simulink model "Pong3D"  (R2016b)
settings: Solver=ode45  StartTime=0.0  StopTime=10.0  FixedStep=0.001  MaxStep=updateFrequency  RelTol=1e-3  EnableMultiTasking=on
values from neighbouring files (symbols this model uses):
  Ball = struct(B_field1,B_value1,B_field2,B_value2,B_field3,B_value3,     B_field4,B_value4,B_field5,B_value5)    [PingPongStructs6DOF.m]
  Contact_Forces = struct(CF_field1,CF_value1,CF_field2,CF_value2,CF_field3,CF_value3)    [PingPongStructs6DOF.m]
  g = 9.81    [PingPongStructs6DOF.m]
  m = V(2)/V(1)    [AIPlayer.m]
  Net = struct(N_field1,N_value1)    [PingPongStructs6DOF.m]
  Robot1 = struct(R1_field1,R1_value1,R1_field2,R1_value2,R1_field3,R1_value3,     R1_field4,R1_value4, R1_field5,R1_value5,R1_field6,R1_value6,     R1_field7,R1_value7,R1_field8,R1_value8,R1_field9,R1_value9,R1_field10,R1_value10,     R1_field11,R1_value11,R1_field12,R1_value12)    [PingPongStructs6DOF.m]
  Robot2 = struct(R2_field1,R2_value1,R2_field2,R2_value2,R2_field3,R2_value3,     R2_field4, R2_value4, R2_field5,R2_value5,R2_field6,R2_value6,     R2_field7, R2_value7, R2_field8, R2_value8, R2_field9, R2_value9, R2_field10, R2_value10,     R2_field11, R2_value11, R2_field12, R2_value12)    [PingPongStructs6DOF.m]
  Table = struct(T_field1,T_value1,T_field2,T_value2)    [PingPongStructs6DOF.m]
undefined symbols (not defined in the file or in its folder): X, Y, Z
libraries: sm_lib x120, nesl_utility x55, fl_lib x48, Contact_Forces_Lib x4, Parts_Lib x3
(part 1 of 5)
settings Model: Creator=philipp  LastModifiedBy=philipp
settings DataIOCC: SaveFormat=Structure
settings OptimizationCC: LifeSpan=inf
settings DebuggingCC: SFUnexpectedBacktrackingDiag=warning  SFNoUnconditionalDefaultTransitionDiag=warning  SFExecutionAtInitializationDiag=none
settings HardwareCC: ProdBitPerSizeT=32  ProdBitPerPtrDiffT=32  ProdWordSize=32  ProdHWDeviceType=Specified
settings GRTTargetCC: TargetLangStandard=C89/C90 (ANSI)  GeneratePreprocessorConditionals=Disable all
settings ConfigComp: CovMetricSettings=dw  CovHtmlReporting=on  CovSaveCumulativeToWorkspaceVar=on  CovSaveSingleToWorkspaceVar=on  CovExternalEMLEnable=off
settings DiagnosticsConfigSet: SimMechanicsRigidlyBoundBlock=warning

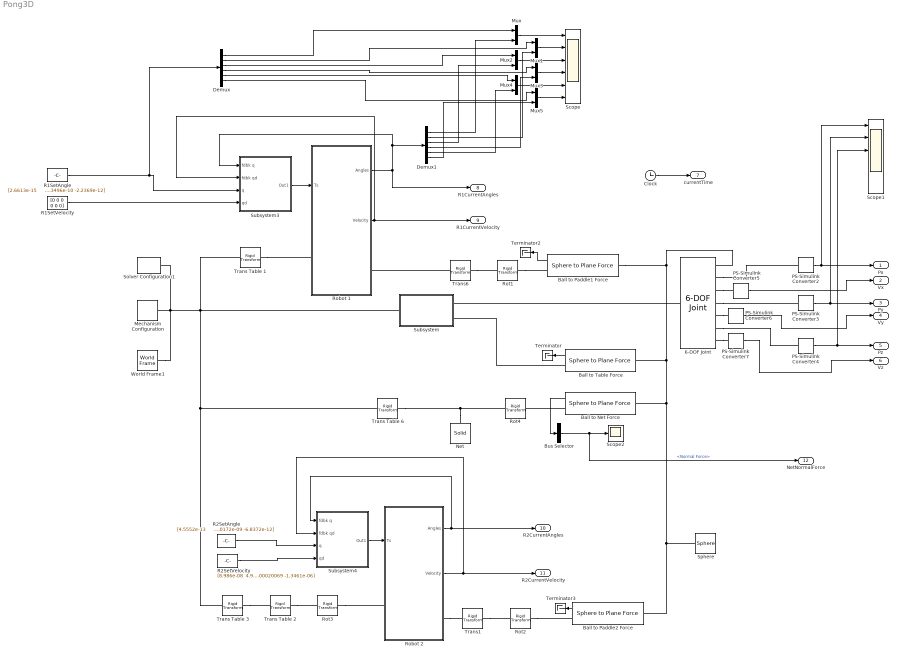
== system Pong3D ==
  6-DOF Joint : sm_lib/Joints/6-DOF Joint  SenseConstraintForce=off  SenseConstraintForceX=off  SenseConstraintForceY=off  SenseConstraintForceZ=off  SenseConstraintTorque=off  SenseConstraintTorqueX=off  SenseConstraintTorqueY=off  SenseConstraintTorqueZ=off  SenseTotalForce=off  SenseTotalForceX=off  SenseTotalForceY=off  SenseTotalForceZ=off  SenseTotalTorque=off  SenseTotalTorqueX=off  SenseTotalTorqueY=off  SenseTotalTorqueZ=off  CompositeWrenchDir=FollowerOnBase  CompositeWrenchFrame=BaseFrame  PxEquilibriumPosition=0  PxEquilibriumPositionUnits=m  PxSpringStiffness=0  PxSpringStiffnessUnits=N/m  PxDampingCoefficient=0  PxDampingCoefficientUnits=N/(m/s)  PxTorqueActuationMode=NoTorque  PxMotionActuationMode=ComputedMotion  PxSensePosition=on  PxSenseVelocity=on  PxSenseAcceleration=off  PxSenseTorqueForce=off  PxPositionTargetSpecify=on  PxPositionTargetPriority=High  PxPositionTargetValue=Ball.Initial_Position(1)  PxPositionTargetValueUnits=m  PxVelocityTargetSpecify=on  PxVelocityTargetPriority=High  PxVelocityTargetValue=Ball.Initial_Velocity(1)  PxVelocityTargetValueUnits=m/s  PyEquilibriumPosition=0  PyEquilibriumPositionUnits=m  PySpringStiffness=0  PySpringStiffnessUnits=N/m  PyDampingCoefficient=0  PyDampingCoefficientUnits=N/(m/s)  PyTorqueActuationMode=NoTorque  PyMotionActuationMode=ComputedMotion  PySensePosition=on  PySenseVelocity=on  PySenseAcceleration=off  PySenseTorqueForce=off  PyPositionTargetSpecify=on  PyPositionTargetPriority=High  PyPositionTargetValue=Ball.Initial_Position(2)  PyPositionTargetValueUnits=m  PyVelocityTargetSpecify=on  PyVelocityTargetPriority=High  PyVelocityTargetValue=Ball.Initial_Velocity(2)  PyVelocityTargetValueUnits=m/s  PzEquilibriumPosition=0  PzEquilibriumPositionUnits=m  PzSpringStiffness=0  PzSpringStiffnessUnits=N/m  PzDampingCoefficient=0  PzDampingCoefficientUnits=N/(m/s)  PzTorqueActuationMode=NoTorque  PzMotionActuationMode=ComputedMotion  PzSensePosition=on  PzSenseVelocity=on  PzSenseAcceleration=off  PzSenseTorqueForce=off  PzPositionTargetSpecify=on  PzPositionTargetPriority=High  PzPositionTargetValue=Ball.Initial_Position(3)  PzPositionTargetValueUnits=m  PzVelocityTargetSpecify=on  PzVelocityTargetPriority=High  PzVelocityTargetValue=Ball.Initial_Velocity(3)  PzVelocityTargetValueUnits=m/s  SphDefPosRotationMethod=None  SphDefPosRotationAngleUnits=deg  SphDefPosRotationStandardAxis=+Z  SphDefPosRotationAngle=0.0  SphDefPosRotationArbitraryAxis=[0 0 1]  SphDefPosFollAlignAxisA=+X  SphDefPosBaseAlignAxisA=+Y  SphDefPosFollAlignAxisB=+Y  SphDefPosBaseAlignAxisB=+Z  SphDefPosRotationSequenceAxes=FollowerAxes  SphDefPosRotationSequence=XYX  SphDefPosRotationSequenceAngles=[0 0 0]  SphDefPosRotationSequenceAnglesUnits=deg  SphDefPosRotationMatrix=[1 0 0; 0 1 0; 0 0 1]  SphEqPosRotationMethod=None  SphEqPosRotationAngleUnits=deg  SphEqPosRotationStandardAxis=+Z  SphEqPosRotationAngle=0.0  SphEqPosRotationArbitraryAxis=[0 0 1]  SphEqPosFollAlignAxisA=+X  SphEqPosBaseAlignAxisA=+Y  SphEqPosFollAlignAxisB=+Y  SphEqPosBaseAlignAxisB=+Z  SphEqPosRotationSequenceAxes=FollowerAxes  SphEqPosRotationSequence=XYX  SphEqPosRotationSequenceAngles=[0 0 0]  SphEqPosRotationSequenceAnglesUnits=deg  SphEqPosRotationMatrix=[1 0 0; 0 1 0; 0 0 1]  SphSpringStiffness=0  SphSpringStiffnessUnits=N*m/deg  SphDampingCoefficient=0  SphDampingCoefficientUnits=N*m/(deg/s)  SphActuateTorqueX=off  SphActuateTorqueY=off  SphActuateTorqueZ=off  SphActuateTorque=off  SphTorqueActuationMode=NoTorque  SphMotionActuationMode=ComputedMotion  SphActuationFrame=BaseFrame  SphSensePosition=off  SphSenseVelocityX=off  SphSenseVelocityY=off  SphSenseVelocityZ=off  SphSenseVelocity=off  SphSenseAccelerationX=off  SphSenseAccelerationY=off  SphSenseAccelerationZ=off  SphSenseAcceleration=off  SphSenseTorqueX=off  SphSenseTorqueY=off  SphSenseTorqueZ=off  SphSenseTorqueForce=off  SphSensingFrame=BaseFrame  SphPositionTargetRotationMethod=None  SphPositionTargetRotationAngleUnits=deg  SphPositionTargetRotationStandardAxis=+Z  SphPositionTargetRotationAngle=0.0  SphPositionTargetRotationArbitraryAxis=[0 0 1]  SphPositionTargetFollAlignAxisA=+X  SphPositionTargetBaseAlignAxisA=+Y  SphPositionTargetFollAlignAxisB=+Y  SphPositionTargetBaseAlignAxisB=+Z  SphPositionTargetRotationSequenceAxes=FollowerAxes  SphPositionTargetRotationSequence=XYX  SphPositionTargetRotationSequenceAngles=[0 0 0]  SphPositionTargetRotationSequenceAnglesUnits=deg  SphPositionTargetRotationMatrix=[1 0 0; 0 1 0; 0 0 1]  SphPositionTargetSpecify=off  SphPositionTargetPriority=High  SphVelocityTargetValue=[0 0 0]  SphVelocityTargetValueUnits=rad/s  SphVelocityTargetSpecify=off  SphVelocityTargetPriority=High  SphVelocityTargetInFollowerFrame=on
  Ball to Net Force : Contact_Forces_Lib/3D/Sphere to Plane Force  sphere_rad=Ball.Radius  plane_lenx=Net.Dimensions(3)  plane_leny=Net.Dimensions(1)  plane_depth=Net.Dimensions(2)/2  force_law=Linear  k_contact=Contact_Forces.Ball_Net(1)  b_contact=Contact_Forces.Ball_Net(2)  pen_full_damp_F=1e-4  pen_exponent=1  custom_param_1=1  custom_param_2=1  friction_law=None  mu_kinetic=0.5  mu_static=0.7  v_thr=0.001
  Ball to Paddle1 Force : Contact_Forces_Lib/3D/Sphere to Plane Force  sphere_rad=Ball.Radius  plane_lenx=2*Robot1.Paddle(1)  plane_leny=2*Robot1.Paddle(1)  plane_depth=Robot1.Paddle(2)/2  force_law=Linear  k_contact=Contact_Forces.Ball_Paddle(1)  b_contact=Contact_Forces.Ball_Paddle(2)  pen_full_damp_F=1e-4  pen_exponent=1  custom_param_1=1  custom_param_2=1  friction_law=None  mu_kinetic=0.5  mu_static=0.7  v_thr=0.001
  Ball to Paddle2 Force : Contact_Forces_Lib/3D/Sphere to Plane Force  sphere_rad=Ball.Radius  plane_lenx=2*Robot2.Paddle(1)  plane_leny=2*Robot2.Paddle(1)  plane_depth=Robot2.Paddle(2)/2  force_law=Linear  k_contact=Contact_Forces.Ball_Paddle(1)  b_contact=Contact_Forces.Ball_Paddle(2)  pen_full_damp_F=1e-4  pen_exponent=1  custom_param_1=1  custom_param_2=1  friction_law=None  mu_kinetic=0.5  mu_static=0.7  v_thr=0.001
  Ball to Table Force : Contact_Forces_Lib/3D/Sphere to Plane Force  sphere_rad=Ball.Radius  plane_lenx=Table.Dimensions(1)  plane_leny=Table.Dimensions(2)  plane_depth=Table.Dimensions(3)/2  force_law=Linear  k_contact=Contact_Forces.Ball_Table(1)  b_contact=Contact_Forces.Ball_Table(2)  pen_full_damp_F=1e-4  pen_exponent=1  custom_param_1=1  custom_param_2=1  friction_law=None  mu_kinetic=0.5  mu_static=0.7  v_thr=0.001
  Bus Selector : BusSelector  OutputSignals=Normal Force
  Clock : Clock
  Demux : Demux  Outputs=6
  Demux1 : Demux  Outputs=6
  Mechanism Configuration : sm_lib/Utilities/Mechanism Configuration  UniformGravity=Constant  GravityVector=[0 0 -g]  GravityUnits=m/s^2  LinearizationDelta=0.001
  Mux{,1..5} (6 alike) : Mux  Inputs=2
  Net : sm_lib/Body Elements/Solid  InertiaType=CalculateFromGeometry  Mass=1  MassUnits=kg  CenterOfMass=[0 0 0]  CenterOfMassUnits=m  MomentsOfInertia=[1 1 1]  MomentsOfInertiaUnits=kg*m^2  ProductsOfInertia=[0 0 0]  ProductsOfInertiaUnits=kg*m^2  DensityBased=on  Density=Net.Dimensions(4)  DensityUnits=kg/(m^3)  DoExposeReferenceFrame=on  SerializedFrames=<Frames/>  GraphicType=FromGeometry  MarkerShape=Sphere  MarkerSize=10  MarkerSizeUnits=m  GraphicVisPropType=SimpleVisualProperties  GraphicDiffuseColor=[1.0 1.0 1.0]  GraphicSpecularColor=[0.5 0.5 0.5 1.0]  GraphicAmbientColor=[0.15 0.15 0.15 1.0]  GraphicEmissiveColor=[0.0 0.0 0.0 1.0]  GraphicShininess=75  GraphicOpacity=1.0  GeometryShape=Brick  RectangleSize=[1 1]  RectangleSizeUnits=m  BrickDimensions=[Net.Dimensions(2) Net.Dimensions(1) Net.Dimensions(3)]  BrickDimensionUnits=m  CylinderRadius=1  CylinderRadiusUnits=m  CylinderLength=1  CylinderLengthUnits=m  SphereRadius=1  SphereRadiusUnits=m  EllipsoidRadii=[1 1 1]  EllipsoidRadiiUnits=m  ExtrusionCrossSection=[1 1; -1 1; -1 -1; 1 -1]  ExtrusionCrossSectionUnits=m  ExtrusionLength=1  ExtrusionLengthUnits=m  PolygonNumSides=3  PolygonOuterRadius=1  PolygonOuterRadiusUnits=m  ExtGeomFileType=STL  ExtGeomFileUnits=m  RevolutionCrossSection=[1 1; 1 -1; 2 -1; 2 1]  RevolutionCrossSectionUnits=m  RevolutionExtent=Full  RevolutionAngle=180  RevolutionAngleUnits=deg
  PS-Simulink Converter{2..7} (6 alike) : nesl_utility/PS-Simulink Converter  PhysicalDomain=network_engine_domain  SubClassName=ps_output  LeftPortType=input  RightPortType=output  PseudoPeriodic=off  Frequencies=[]  Unit=1  AffineConversion=off
  R1SetAngle : Constant  Value="[2.6613e-15      1.5708 -1.8519e-10  2.2643e-12  3.3496e-10 -2.2369e-12]"
  R1SetVelocity : Constant  Value="[0  0  0  0  0  0]"
  R2SetAngle : Constant  Value="[4.5552e-13      1.5708  -5.714e-10  6.9506e-12  1.0172e-09 -6.8372e-12]"
  R2SetVelocity : Constant  Value="[8.986e-08  4.9161e-06 -0.00011274  1.3713e-06  0.00020069 -1.3461e-06]"
  Robot 1 : Subsystem
  Robot 2 : Subsystem
  Rot1 : sm_lib/Frames and Transforms/Rigid Transform  TranslationMethod=None  TranslationStandardOffset=0  TranslationLengthUnit=m  TranslationStandardAxis=+Z  TranslationCartesianOffset=[0 0 0]  TranslationROffset=0  TranslationROffsetUnits=m  TranslationZOffset=0  TranslationZOffsetUnits=m  TranslationThetaOffset=0  TranslationThetaOffsetUnits=deg  RotationMethod=StandardAxis  RotationAngleUnits=deg  RotationStandardAxis=-Y  RotationAngle=90  RotationArbitraryAxis=[0 0 1]  FollAlignAxisA=+X  BaseAlignAxisA=+Y  FollAlignAxisB=+Y  BaseAlignAxisB=+Z  RotationSequenceAxes=FollowerAxes  RotationSequence=XYX  RotationSequenceAngles=[0 0 0]  RotationSequenceAnglesUnits=deg  RotationMatrix=[1 0 0; 0 1 0; 0 0 1]
      settings: AttributesFormatString=|
      | %<RotationAngle> %<RotationAngleUnits>
      | about %<RotationStandardAxis>
  Rot2 : sm_lib/Frames and Transforms/Rigid Transform  TranslationMethod=None  TranslationStandardOffset=0  TranslationLengthUnit=m  TranslationStandardAxis=+Z  TranslationCartesianOffset=[0 0 0]  TranslationROffset=0  TranslationROffsetUnits=m  TranslationZOffset=0  TranslationZOffsetUnits=m  TranslationThetaOffset=0  TranslationThetaOffsetUnits=deg  RotationMethod=StandardAxis  RotationAngleUnits=deg  RotationStandardAxis=-Y  RotationAngle=90  RotationArbitraryAxis=[0 0 1]  FollAlignAxisA=+X  BaseAlignAxisA=+Y  FollAlignAxisB=+Y  BaseAlignAxisB=+Z  RotationSequenceAxes=FollowerAxes  RotationSequence=XYX  RotationSequenceAngles=[0 0 0]  RotationSequenceAnglesUnits=deg  RotationMatrix=[1 0 0; 0 1 0; 0 0 1]
      settings: AttributesFormatString=|
      | %<RotationAngle> %<RotationAngleUnits>
      | about %<RotationStandardAxis>
  Rot3 : sm_lib/Frames and Transforms/Rigid Transform  TranslationMethod=None  TranslationStandardOffset=0  TranslationLengthUnit=m  TranslationStandardAxis=+Z  TranslationCartesianOffset=[0 0 0]  TranslationROffset=0  TranslationROffsetUnits=m  TranslationZOffset=0  TranslationZOffsetUnits=m  TranslationThetaOffset=0  TranslationThetaOffsetUnits=deg  RotationMethod=StandardAxis  RotationAngleUnits=deg  RotationStandardAxis=+Z  RotationAngle=180  RotationArbitraryAxis=[0 0 1]  FollAlignAxisA=+X  BaseAlignAxisA=+Y  FollAlignAxisB=+Y  BaseAlignAxisB=+Z  RotationSequenceAxes=FollowerAxes  RotationSequence=XYX  RotationSequenceAngles=[0 0 0]  RotationSequenceAnglesUnits=deg  RotationMatrix=[1 0 0; 0 1 0; 0 0 1]
      settings: AttributesFormatString=|
      | %<RotationAngle> %<RotationAngleUnits>
      | about %<RotationStandardAxis>
  Rot4 : sm_lib/Frames and Transforms/Rigid Transform  TranslationMethod=None  TranslationStandardOffset=0  TranslationLengthUnit=m  TranslationStandardAxis=+Z  TranslationCartesianOffset=[0 0 0]  TranslationROffset=0  TranslationROffsetUnits=m  TranslationZOffset=0  TranslationZOffsetUnits=m  TranslationThetaOffset=0  TranslationThetaOffsetUnits=deg  RotationMethod=StandardAxis  RotationAngleUnits=deg  RotationStandardAxis=-Y  RotationAngle=90  RotationArbitraryAxis=[0 0 1]  FollAlignAxisA=+X  BaseAlignAxisA=+Y  FollAlignAxisB=+Y  BaseAlignAxisB=+Z  RotationSequenceAxes=FollowerAxes  RotationSequence=XYX  RotationSequenceAngles=[0 0 0]  RotationSequenceAnglesUnits=deg  RotationMatrix=[1 0 0; 0 1 0; 0 0 1]
      settings: AttributesFormatString=|
      | %<RotationAngle> %<RotationAngleUnits>
      | about %<RotationStandardAxis>
  Scope : Scope  NumInputPorts=6
  Scope1 : Scope  NumInputPorts=6
  Scope2 : Scope
  Solver Configuration1 : nesl_utility/Solver Configuration  PhysicalDomain=network_engine_domain  SubClassName=solver  LeftPortType=input  RightPortType=generic  Accelerate=off  Tones=[]  Harmonics=[]  SimulateNoise=off  Profile=off  UseLocalSampling=off  EnableSwitchedLinearOptims=on  FrequencyDomain=off  UseCCode=off  RelTol=0.001  AbsTol=1e-06  MinStep=1e-09  ToWorkspace=off  RevertToSquareIcSolve=off  NumHomotopyIterations=100  PhasorMode=off  PhasorModeNumHarmonics=1  OverrideAbsTol=off  DoDC=off  ResidualTolerance=1e-09  UseLocalSolver=off  LocalSolverChoice=NE_BACKWARD_EULER_ADVANCER  LocalSolverSampleTime=0.001  DoFixedCost=off  MaxNonlinIter=3  MaxModeIter=2  LinearAlgebra=Sparse  DelaysMemoryBudget=1024  AutomaticFiltering=on  FilteringTimeConstant=0.001
  Sphere : Parts_Lib/Sphere  Tag=CustomStyle  sph_radius=Ball.Radius  sph_density=Ball.Density  sph_color=white  sph_opacity=1  mark_type=Rings on center planes  arc_width=[40 50]  arc_angle=60  ring_width=5  ring_irad=0.95  mark_color=axes  mark_opacity=1  ring_opacity=0  arc_opacity=0
  Subsystem : Subsystem
  Subsystem3 : Subsystem
  Subsystem4 : Subsystem
  Terminator : Terminator
  Terminator2 : Terminator
  Terminator3 : Terminator
  Trans Table 1 : sm_lib/Frames and Transforms/Rigid Transform  TranslationMethod=StandardAxis  TranslationStandardOffset=-Table.Dimensions(1)/2-Robot1.Distance_Table(1)  TranslationLengthUnit=m  TranslationStandardAxis=+X  TranslationCartesianOffset=[0 0 0]  TranslationROffset=0  TranslationROffsetUnits=m  TranslationZOffset=0  TranslationZOffsetUnits=m  TranslationThetaOffset=0  TranslationThetaOffsetUnits=deg  RotationMethod=None  RotationAngleUnits=deg  RotationStandardAxis=+Z  RotationAngle=0.0  RotationArbitraryAxis=[0 0 1]  FollAlignAxisA=+X  BaseAlignAxisA=+Y  FollAlignAxisB=+Y  BaseAlignAxisB=+Z  RotationSequenceAxes=FollowerAxes  RotationSequence=XYX  RotationSequenceAngles=[0 0 0]  RotationSequenceAnglesUnits=deg  RotationMatrix=[1 0 0; 0 1 0; 0 0 1]
      settings: AttributesFormatString=|
      | %<TranslationStandardOffset> %<TranslationLengthUnit>
      | in %<TranslationStandardAxis>
  Trans Table 2 : sm_lib/Frames and Transforms/Rigid Transform  TranslationMethod=StandardAxis  TranslationStandardOffset=-Table.Dimensions(1)/2-Robot1.Distance_Table(1)  TranslationLengthUnit=m  TranslationStandardAxis=+X  TranslationCartesianOffset=[0 0 0]  TranslationROffset=0  TranslationROffsetUnits=m  TranslationZOffset=0  TranslationZOffsetUnits=m  TranslationThetaOffset=0  TranslationThetaOffsetUnits=deg  RotationMethod=None  RotationAngleUnits=deg  RotationStandardAxis=+Z  RotationAngle=0.0  RotationArbitraryAxis=[0 0 1]  FollAlignAxisA=+X  BaseAlignAxisA=+Y  FollAlignAxisB=+Y  BaseAlignAxisB=+Z  RotationSequenceAxes=FollowerAxes  RotationSequence=XYX  RotationSequenceAngles=[0 0 0]  RotationSequenceAnglesUnits=deg  RotationMatrix=[1 0 0; 0 1 0; 0 0 1]
      settings: AttributesFormatString=|
      | %<TranslationStandardOffset> %<TranslationLengthUnit>
      | in %<TranslationStandardAxis>
  Trans Table 3 : sm_lib/Frames and Transforms/Rigid Transform  TranslationMethod=StandardAxis  TranslationStandardOffset=Table.Dimensions(1)+Robot1.Distance_Table(1)+Robot2.Distance_Table(1)  TranslationLengthUnit=m  TranslationStandardAxis=+X  TranslationCartesianOffset=[0 0 0]  TranslationROffset=0  TranslationROffsetUnits=m  TranslationZOffset=0  TranslationZOffsetUnits=m  TranslationThetaOffset=0  TranslationThetaOffsetUnits=deg  RotationMethod=None  RotationAngleUnits=deg  RotationStandardAxis=+Z  RotationAngle=0.0  RotationArbitraryAxis=[0 0 1]  FollAlignAxisA=+X  BaseAlignAxisA=+Y  FollAlignAxisB=+Y  BaseAlignAxisB=+Z  RotationSequenceAxes=FollowerAxes  RotationSequence=XYX  RotationSequenceAngles=[0 0 0]  RotationSequenceAnglesUnits=deg  RotationMatrix=[1 0 0; 0 1 0; 0 0 1]
      settings: AttributesFormatString=|
      | %<TranslationStandardOffset> %<TranslationLengthUnit>
      | in %<TranslationStandardAxis>
  Trans Table 6 : sm_lib/Frames and Transforms/Rigid Transform  TranslationMethod=StandardAxis  TranslationStandardOffset=Table.Height+Net.Dimensions(3)/2  TranslationLengthUnit=m  TranslationStandardAxis=+Z  TranslationCartesianOffset=[0 0 0]  TranslationROffset=0  TranslationROffsetUnits=m  TranslationZOffset=0  TranslationZOffsetUnits=m  TranslationThetaOffset=0  TranslationThetaOffsetUnits=deg  RotationMethod=None  RotationAngleUnits=deg  RotationStandardAxis=+Z  RotationAngle=0.0  RotationArbitraryAxis=[0 0 1]  FollAlignAxisA=+X  BaseAlignAxisA=+Y  FollAlignAxisB=+Y  BaseAlignAxisB=+Z  RotationSequenceAxes=FollowerAxes  RotationSequence=XYX  RotationSequenceAngles=[0 0 0]  RotationSequenceAnglesUnits=deg  RotationMatrix=[1 0 0; 0 1 0; 0 0 1]
      settings: AttributesFormatString=|
      | %<TranslationStandardOffset> %<TranslationLengthUnit>
      | in %<TranslationStandardAxis>
  Trans1 : sm_lib/Frames and Transforms/Rigid Transform  TranslationMethod=StandardAxis  TranslationStandardOffset=Robot2.Paddle(1)  TranslationLengthUnit=m  TranslationStandardAxis=-Z  TranslationCartesianOffset=[0 0 0]  TranslationROffset=0  TranslationROffsetUnits=m  TranslationZOffset=0  TranslationZOffsetUnits=m  TranslationThetaOffset=0  TranslationThetaOffsetUnits=deg  RotationMethod=None  RotationAngleUnits=deg  RotationStandardAxis=+Z  RotationAngle=0.0  RotationArbitraryAxis=[0 0 1]  FollAlignAxisA=+X  BaseAlignAxisA=+Y  FollAlignAxisB=+Y  BaseAlignAxisB=+Z  RotationSequenceAxes=FollowerAxes  RotationSequence=XYX  RotationSequenceAngles=[0 0 0]  RotationSequenceAnglesUnits=deg  RotationMatrix=[1 0 0; 0 1 0; 0 0 1]
      settings: AttributesFormatString=|
      | %<TranslationStandardOffset> %<TranslationLengthUnit>
      | in %<TranslationStandardAxis>
  Trans6 : sm_lib/Frames and Transforms/Rigid Transform  TranslationMethod=StandardAxis  TranslationStandardOffset=Robot1.Paddle(1)  TranslationLengthUnit=m  TranslationStandardAxis=-Z  TranslationCartesianOffset=[0 0 0]  TranslationROffset=0  TranslationROffsetUnits=m  TranslationZOffset=0  TranslationZOffsetUnits=m  TranslationThetaOffset=0  TranslationThetaOffsetUnits=deg  RotationMethod=None  RotationAngleUnits=deg  RotationStandardAxis=+Z  RotationAngle=0.0  RotationArbitraryAxis=[0 0 1]  FollAlignAxisA=+X  BaseAlignAxisA=+Y  FollAlignAxisB=+Y  BaseAlignAxisB=+Z  RotationSequenceAxes=FollowerAxes  RotationSequence=XYX  RotationSequenceAngles=[0 0 0]  RotationSequenceAnglesUnits=deg  RotationMatrix=[1 0 0; 0 1 0; 0 0 1]
      settings: AttributesFormatString=|
      | %<TranslationStandardOffset> %<TranslationLengthUnit>
      | in %<TranslationStandardAxis>
  World Frame1 : sm_lib/Frames and Transforms/World Frame
  Px : Outport
  Vx : Outport  Port=2
  Py : Outport  Port=3
  Vy : Outport  Port=4
  Pz : Outport  Port=5
  Vz : Outport  Port=6
  currentTime : Outport  Port=7
  R1CurrentAngles : Outport  Port=8  PortDimensions=[1,6]
  R1CurrentVelocity : Outport  Port=9  PortDimensions=[1,6]
  R2CurrentAngles : Outport  Port=10  PortDimensions=[1,6]
  R2CurrentVelocity : Outport  Port=11  PortDimensions=[1,6]
  NetNormalForce : Outport  Port=12
  wires:
  Subsystem3/1(Out1) -> Robot 1/1(Ts)
  Subsystem4/1(Out1) -> Robot 2/1(Ts)
  Ball to Table Force/1 -> Terminator/1
  Ball to Net Force/1 -> Bus Selector/1
  Ball to Paddle1 Force/1 -> Terminator2/1
  Ball to Paddle2 Force/1 -> Terminator3/1
  PS-Simulink Converter2/1 -> Px/1, Scope1/1
  PS-Simulink Converter4/1 -> Scope1/3, Pz/1
  PS-Simulink Converter3/1 -> Py/1, Scope1/2
  PS-Simulink Converter6/1 -> Vy/1
  PS-Simulink Converter5/1 -> Vx/1
  PS-Simulink Converter7/1 -> Vz/1
  R1SetAngle/1 -> Demux/1, Subsystem3/3(q)
  Mux/1 -> Scope/1
  Mux1/1 -> Scope/2
  Mux2/1 -> Scope/3
  Mux3/1 -> Scope/4
  Mux4/1 -> Scope/5
  Demux/5 -> Mux4/1
  Mux5/1 -> Scope/6
  Demux/1 -> Mux/1
  Demux/2 -> Mux1/1
  Demux/3 -> Mux2/1
  Demux/4 -> Mux3/1
  Demux/6 -> Mux5/1
  Demux1/1 -> Mux/2
  Demux1/2 -> Mux1/2
  Demux1/3 -> Mux2/2
  Demux1/4 -> Mux3/2
  Demux1/5 -> Mux4/2
  Demux1/6 -> Mux5/2
  R2SetAngle/1 -> Subsystem4/3(q)
  R1SetVelocity/1 -> Subsystem3/4(qd)
  R2SetVelocity/1 -> Subsystem4/4(qd)
  Robot 1/2(Velocity) -> Subsystem3/2(fdbk qd), R1CurrentVelocity/1
  Robot 1/1(Angles) -> R1CurrentAngles/1, Demux1/1, Subsystem3/1(fdbk q)
  Robot 2/1(Angles) -> Subsystem4/1(fdbk q), R2CurrentAngles/1
  Robot 2/2(Velocity) -> Subsystem4/2(fdbk qd), R2CurrentVelocity/1
  Bus Selector/1 -> NetNormalForce/1, Scope2/1  "<Normal Force>"
  Clock/1 -> currentTime/1
  connections:
  Net/RConn1 -- Rot4/LConn1 -- Trans Table 6/RConn1
  6-DOF Joint/LConn1 -- Subsystem/RConn1
  World Frame1/RConn1 -- Subsystem/LConn1 -- Trans Table 1/LConn1 -- Trans Table 6/LConn1 -- Trans Table 3/LConn1 -- Solver Configuration1/RConn1 -- Mechanism Configuration/RConn1
  Ball to Table Force/RConn1 -- Subsystem/RConn2
  Ball to Paddle2 Force/LConn1 -- Ball to Paddle1 Force/LConn1 -- 6-DOF Joint/RConn1 -- Ball to Table Force/LConn1 -- Ball to Net Force/LConn1 -- Sphere/LConn1
  Trans6/LConn1 -- Robot 1/RConn1
  Robot 2/RConn1 -- Trans1/LConn1
  Rot3/RConn1 -- Robot 2/LConn1
  Trans Table 3/RConn1 -- Trans Table 2/LConn1
  6-DOF Joint/RConn2 -- PS-Simulink Converter2/LConn1
  6-DOF Joint/RConn3 -- PS-Simulink Converter5/LConn1
  6-DOF Joint/RConn4 -- PS-Simulink Converter3/LConn1
  6-DOF Joint/RConn6 -- PS-Simulink Converter4/LConn1
  6-DOF Joint/RConn5 -- PS-Simulink Converter6/LConn1
  6-DOF Joint/RConn7 -- PS-Simulink Converter7/LConn1
  Rot1/RConn1 -- Ball to Paddle1 Force/RConn1
  Trans6/RConn1 -- Rot1/LConn1
  Rot2/RConn1 -- Ball to Paddle2 Force/RConn1
  Trans1/RConn1 -- Rot2/LConn1
  Trans Table 1/RConn1 -- Robot 1/LConn1
  Trans Table 2/RConn1 -- Rot3/LConn1
  Ball to Net Force/RConn1 -- Rot4/RConn1

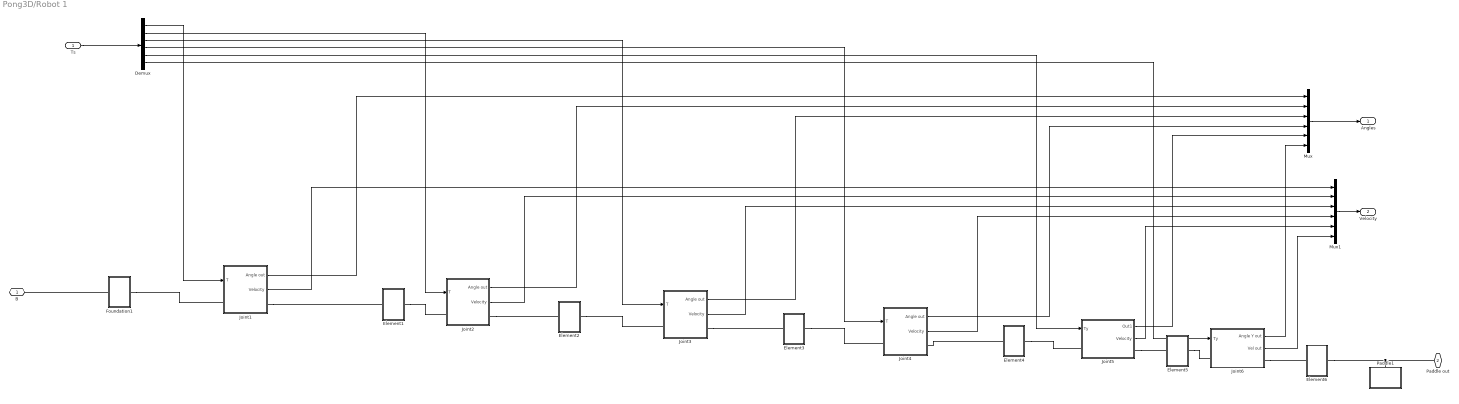
== system Pong3D/Robot 1 ==
  Ts : Inport
  Demux : Demux  Outputs=6
  Element1 : Subsystem
  Element2 : Subsystem
  Element3 : Subsystem
  Element4 : Subsystem
  Element5 : Subsystem
  Element6 : Subsystem
  Foundation1 : Subsystem
  Joint1 : Subsystem
  Joint2 : Subsystem
  Joint3 : Subsystem
  Joint4 : Subsystem
  Joint5 : Subsystem
  Joint6 : Subsystem
  Mux : Mux  Inputs=6
  Mux1 : Mux  Inputs=6
  Paddle1 : Subsystem
  B : PMIOPort  Port=1  Side=Left
  Paddle out : PMIOPort  Port=2  Side=Right
  Angles : Outport
  Velocity : Outport  Port=2
  wires:
  Joint6/1(Angle Y out) -> Mux/6
  Joint5/1(Out1) -> Mux/5
  Joint4/1(Angle out) -> Mux/4
  Joint3/1(Angle out) -> Mux/3
  Joint2/1(Angle out) -> Mux/2
  Joint1/1(Angle out) -> Mux/1
  Ts/1 -> Demux/1
  Demux/1 -> Joint1/1(T)
  Demux/2 -> Joint2/1(T)
  Demux/3 -> Joint3/1(T)
  Demux/4 -> Joint4/1(T)
  Demux/5 -> Joint5/1(Ty)
  Demux/6 -> Joint6/1(Ty)
  Joint6/2(Vel out) -> Mux1/6
  Mux/1 -> Angles/1
  Mux1/1 -> Velocity/1
  Joint5/2(Velocity) -> Mux1/5
  Joint4/2(Velocity) -> Mux1/4
  Joint3/2(Velocity) -> Mux1/3
  Joint2/2(Velocity) -> Mux1/2
  Joint1/2(Velocity) -> Mux1/1
  connections:
  Joint4/RConn1 -- Element4/LConn1
  Element3/RConn1 -- Joint4/LConn1
  Joint2/RConn1 -- Element2/LConn1
  Element1/RConn1 -- Joint2/LConn1
  Foundation1/RConn1 -- Joint1/LConn1
  Joint3/RConn1 -- Element3/LConn1
  Element4/RConn1 -- Joint5/LConn1
  Element5/RConn1 -- Joint6/LConn1
  Joint6/RConn1 -- Element6/LConn1
  Foundation1/LConn1 -- B/RConn1
  Joint1/RConn1 -- Element1/LConn1
  Element2/RConn1 -- Joint3/LConn1
  Joint5/RConn1 -- Element5/LConn1
  Element6/RConn1 -- Paddle out/RConn1 -- Paddle1/LConn1

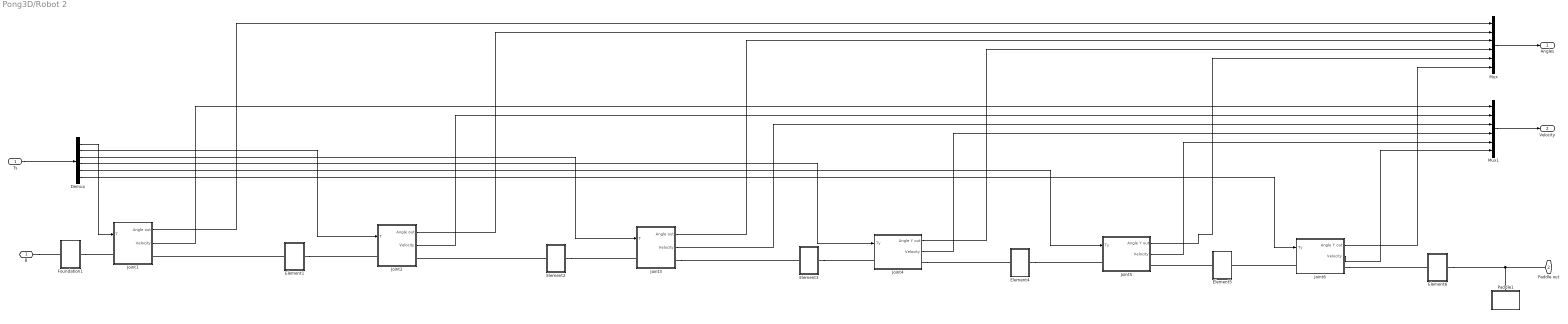
== system Pong3D/Robot 2 ==
  Ts : Inport
  Demux : Demux  Outputs=6
  Element1 : Subsystem
  Element2 : Subsystem
  Element3 : Subsystem
  Element4 : Subsystem
  Element5 : Subsystem
  Element6 : Subsystem
  Foundation1 : Subsystem
  Joint1 : Subsystem
  Joint2 : Subsystem
  Joint3 : Subsystem
  Joint4 : Subsystem
  Joint5 : Subsystem
  Joint6 : Subsystem
  Mux : Mux  Inputs=6
  Mux1 : Mux  Inputs=6
  Paddle1 : Subsystem
  B : PMIOPort  Port=1  Side=Left
  Paddle out : PMIOPort  Port=2  Side=Right
  Angles : Outport
  Velocity : Outport  Port=2
  wires:
  Ts/1 -> Demux/1
  Demux/1 -> Joint1/1(T)
  Demux/2 -> Joint2/1(T)
  Demux/3 -> Joint3/1(T)
  Demux/4 -> Joint4/1(Ty)
  Demux/5 -> Joint5/1(Ty)
  Demux/6 -> Joint6/1(Ty)
  Mux/1 -> Angles/1
  Joint6/1(Angle Y out) -> Mux/6
  Joint5/1(Angle Y out) -> Mux/5
  Joint4/1(Angle Y out) -> Mux/4
  Joint3/1(Angle out) -> Mux/3
  Joint2/1(Angle out) -> Mux/2
  Joint1/1(Angle out) -> Mux/1
  Mux1/1 -> Velocity/1
  Joint6/2(Velocity) -> Mux1/6
  Joint5/2(Velocity) -> Mux1/5
  Joint4/2(Velocity) -> Mux1/4
  Joint3/2(Velocity) -> Mux1/3
  Joint2/2(Velocity) -> Mux1/2
  Joint1/2(Velocity) -> Mux1/1
  connections:
  Element2/LConn1 -- Joint2/RConn1
  Element4/RConn1 -- Joint5/LConn1
  Element1/RConn1 -- Joint2/LConn1
  Element2/RConn1 -- Joint3/LConn1
  Element3/RConn1 -- Joint4/LConn1
  Element5/LConn1 -- Joint5/RConn1
  Element1/LConn1 -- Joint1/RConn1
  B/RConn1 -- Foundation1/LConn1
  Foundation1/RConn1 -- Joint1/LConn1
  Joint3/RConn1 -- Element3/LConn1
  Joint4/RConn1 -- Element4/LConn1
  Paddle out/RConn1 -- Element6/RConn1 -- Paddle1/LConn1
  Joint6/LConn1 -- Element5/RConn1
  Joint6/RConn1 -- Element6/LConn1

== system Pong3D/Subsystem ==
  Table : sm_lib/Body Elements/Solid  InertiaType=CalculateFromGeometry  Mass=1  MassUnits=kg  CenterOfMass=[0 0 0]  CenterOfMassUnits=m  MomentsOfInertia=[1 1 1]  MomentsOfInertiaUnits=kg*m^2  ProductsOfInertia=[0 0 0]  ProductsOfInertiaUnits=kg*m^2  DensityBased=on  Density=Table.Dimensions(4)  DensityUnits=kg/(m^3)  DoExposeReferenceFrame=on  SerializedFrames=<Frames/>  GraphicType=FromGeometry  MarkerShape=Sphere  MarkerSize=10  MarkerSizeUnits=m  GraphicVisPropType=SimpleVisualProperties  GraphicDiffuseColor=[0.0 0.4 0.4]  GraphicSpecularColor=[0.5 0.5 0.5 1.0]  GraphicAmbientColor=[0.15 0.15 0.15 1.0]  GraphicEmissiveColor=[0.0 0.0 0.0 1.0]  GraphicShininess=75  GraphicOpacity=1.0  GeometryShape=Brick  RectangleSize=[1 1]  RectangleSizeUnits=m  BrickDimensions=[Table.Dimensions(1) Table.Dimensions(2) Table.Dimensions(3)]  BrickDimensionUnits=m  CylinderRadius=0.05  CylinderRadiusUnits=m  CylinderLength=0.5  CylinderLengthUnits=m  SphereRadius=1  SphereRadiusUnits=m  EllipsoidRadii=[1 1 1]  EllipsoidRadiiUnits=m  ExtrusionCrossSection=[1 1; -1 1; -1 -1; 1 -1]  ExtrusionCrossSectionUnits=m  ExtrusionLength=1  ExtrusionLengthUnits=m  PolygonNumSides=3  PolygonOuterRadius=1  PolygonOuterRadiusUnits=m  ExtGeomFileType=STL  ExtGeomFileUnits=m  RevolutionCrossSection=[1 1; 1 -1; 2 -1; 2 1]  RevolutionCrossSectionUnits=m  RevolutionExtent=Full  RevolutionAngle=180  RevolutionAngleUnits=deg
  Trans Table 3 : sm_lib/Frames and Transforms/Rigid Transform  TranslationMethod=StandardAxis  TranslationStandardOffset=Table.Height-Table.Dimensions(3)/2  TranslationLengthUnit=m  TranslationStandardAxis=+Z  TranslationCartesianOffset=[0 0 0]  TranslationROffset=0  TranslationROffsetUnits=m  TranslationZOffset=0  TranslationZOffsetUnits=m  TranslationThetaOffset=0  TranslationThetaOffsetUnits=deg  RotationMethod=None  RotationAngleUnits=deg  RotationStandardAxis=+Z  RotationAngle=0.0  RotationArbitraryAxis=[0 0 1]  FollAlignAxisA=+X  BaseAlignAxisA=+Y  FollAlignAxisB=+Y  BaseAlignAxisB=+Z  RotationSequenceAxes=FollowerAxes  RotationSequence=XYX  RotationSequenceAngles=[0 0 0]  RotationSequenceAnglesUnits=deg  RotationMatrix=[1 0 0; 0 1 0; 0 0 1]
      settings: AttributesFormatString=|
      | %<TranslationStandardOffset> %<TranslationLengthUnit>
      | in %<TranslationStandardAxis>
  In : PMIOPort  Port=1  Side=Left
  Bottom : PMIOPort  Port=2  Side=Right
  Center_Table : PMIOPort  Port=3  Side=Right
  connections:
  Center_Table/RConn1 -- Trans Table 3/RConn1 -- Table/RConn1
  Bottom/RConn1 -- In/RConn1 -- Trans Table 3/LConn1

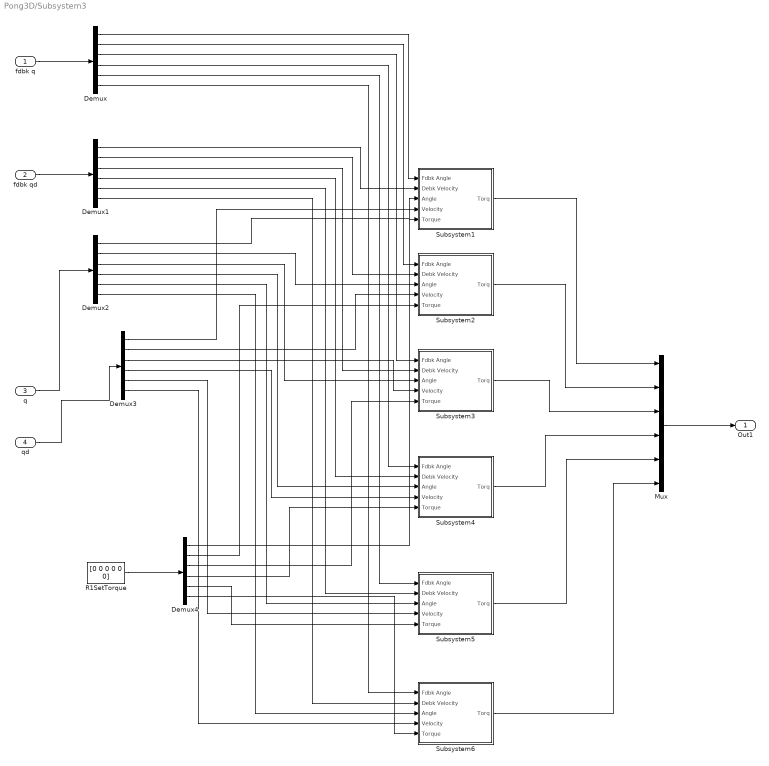
== system Pong3D/Subsystem3 ==
  fdbk q : Inport
  fdbk qd : Inport  Port=2
  q : Inport  Port=3
  qd : Inport  Port=4
  Demux{,1..4} (5 alike) : Demux  Outputs=6
  Mux : Mux  Inputs=6
  R1SetTorque : Constant  Value=[0 0 0 0 0 0]
  Subsystem1 : Subsystem
  Subsystem2 : Subsystem
  Subsystem3 : Subsystem
  Subsystem4 : Subsystem
  Subsystem5 : Subsystem
  Subsystem6 : Subsystem
  Out1 : Outport
  wires:
  q/1 -> Demux2/1
  qd/1 -> Demux3/1
  fdbk q/1 -> Demux/1
  Demux/1 -> Subsystem1/1(Fdbk Angle)
  Demux/2 -> Subsystem2/1(Fdbk Angle)
  Demux/3 -> Subsystem3/1(Fdbk Angle)
  Demux/4 -> Subsystem4/1(Fdbk Angle)
  Demux/5 -> Subsystem5/1(Fdbk Angle)
  Demux/6 -> Subsystem6/1(Fdbk Angle)
  fdbk qd/1 -> Demux1/1
  Demux1/1 -> Subsystem1/2(Debk Velocity)
  Demux1/2 -> Subsystem2/2(Debk Velocity)
  Demux1/3 -> Subsystem3/2(Debk Velocity)
  Demux1/4 -> Subsystem4/2(Debk Velocity)
  Demux1/5 -> Subsystem5/2(Debk Velocity)
  Demux1/6 -> Subsystem6/2(Debk Velocity)
  Demux2/1 -> Subsystem1/3(Angle)
  Demux2/2 -> Subsystem2/3(Angle)
  Demux2/3 -> Subsystem3/3(Angle)
  Demux2/4 -> Subsystem4/3(Angle)
  Demux2/5 -> Subsystem5/3(Angle)
  Demux2/6 -> Subsystem6/3(Angle)
  Demux3/1 -> Subsystem1/4(Velocity)
  Demux3/2 -> Subsystem2/4(Velocity)
  Demux3/3 -> Subsystem3/4(Velocity)
  Demux3/4 -> Subsystem4/4(Velocity)
  Demux3/5 -> Subsystem5/4(Velocity)
  Demux3/6 -> Subsystem6/4(Velocity)
  Demux4/1 -> Subsystem1/5(Torque)
  Demux4/2 -> Subsystem2/5(Torque)
  Demux4/3 -> Subsystem3/5(Torque)
  Demux4/4 -> Subsystem4/5(Torque)
  Demux4/5 -> Subsystem5/5(Torque)
  Demux4/6 -> Subsystem6/5(Torque)
  Subsystem1/1(Torq) -> Mux/1
  Subsystem2/1(Torq) -> Mux/2
  Subsystem3/1(Torq) -> Mux/3
  Subsystem4/1(Torq) -> Mux/4
  Subsystem5/1(Torq) -> Mux/5
  Subsystem6/1(Torq) -> Mux/6
  Mux/1 -> Out1/1
  R1SetTorque/1 -> Demux4/1

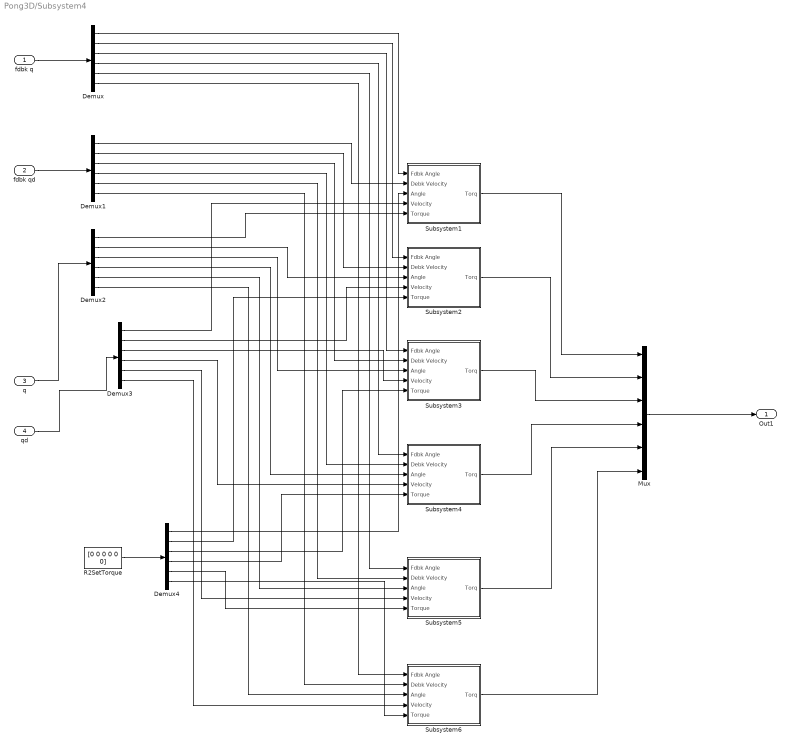
== system Pong3D/Subsystem4 ==
  fdbk q : Inport
  fdbk qd : Inport  Port=2
  q : Inport  Port=3
  qd : Inport  Port=4
  Demux{,1..4} (5 alike) : Demux  Outputs=6
  Mux : Mux  Inputs=6
  R2SetTorque : Constant  Value=[0 0 0 0 0 0]
  Subsystem1 : Subsystem
  Subsystem2 : Subsystem
  Subsystem3 : Subsystem
  Subsystem4 : Subsystem
  Subsystem5 : Subsystem
  Subsystem6 : Subsystem
  Out1 : Outport
  wires:
  Mux/1 -> Out1/1
  Subsystem6/1(Torq) -> Mux/6
  Subsystem5/1(Torq) -> Mux/5
  Subsystem4/1(Torq) -> Mux/4
  Subsystem3/1(Torq) -> Mux/3
  Subsystem2/1(Torq) -> Mux/2
  Subsystem1/1(Torq) -> Mux/1
  Demux4/6 -> Subsystem6/5(Torque)
  Demux4/5 -> Subsystem5/5(Torque)
  Demux4/4 -> Subsystem4/5(Torque)
  Demux4/3 -> Subsystem3/5(Torque)
  Demux4/2 -> Subsystem2/5(Torque)
  Demux4/1 -> Subsystem1/5(Torque)
  Demux3/6 -> Subsystem6/4(Velocity)
  Demux3/5 -> Subsystem5/4(Velocity)
  Demux3/4 -> Subsystem4/4(Velocity)
  Demux3/3 -> Subsystem3/4(Velocity)
  Demux3/2 -> Subsystem2/4(Velocity)
  Demux3/1 -> Subsystem1/4(Velocity)
  Demux2/6 -> Subsystem6/3(Angle)
  Demux2/5 -> Subsystem5/3(Angle)
  Demux2/4 -> Subsystem4/3(Angle)
  Demux2/3 -> Subsystem3/3(Angle)
  Demux2/2 -> Subsystem2/3(Angle)
  Demux2/1 -> Subsystem1/3(Angle)
  Demux1/6 -> Subsystem6/2(Debk Velocity)
  Demux1/5 -> Subsystem5/2(Debk Velocity)
  Demux1/4 -> Subsystem4/2(Debk Velocity)
  Demux1/3 -> Subsystem3/2(Debk Velocity)
  Demux1/2 -> Subsystem2/2(Debk Velocity)
  Demux1/1 -> Subsystem1/2(Debk Velocity)
  fdbk qd/1 -> Demux1/1
  Demux/6 -> Subsystem6/1(Fdbk Angle)
  Demux/5 -> Subsystem5/1(Fdbk Angle)
  Demux/4 -> Subsystem4/1(Fdbk Angle)
  Demux/3 -> Subsystem3/1(Fdbk Angle)
  Demux/2 -> Subsystem2/1(Fdbk Angle)
  Demux/1 -> Subsystem1/1(Fdbk Angle)
  fdbk q/1 -> Demux/1
  qd/1 -> Demux3/1
  q/1 -> Demux2/1
  R2SetTorque/1 -> Demux4/1

== system Pong3D/Robot 1/Element1 ==
  Rot1 : sm_lib/Frames and Transforms/Rigid Transform  TranslationMethod=None  TranslationStandardOffset=0  TranslationLengthUnit=m  TranslationStandardAxis=+Z  TranslationCartesianOffset=[0 0 0]  TranslationROffset=0  TranslationROffsetUnits=m  TranslationZOffset=0  TranslationZOffsetUnits=m  TranslationThetaOffset=0  TranslationThetaOffsetUnits=deg  RotationMethod=StandardAxis  RotationAngleUnits=deg  RotationStandardAxis=-Y  RotationAngle=90  RotationArbitraryAxis=[0 0 1]  FollAlignAxisA=+X  BaseAlignAxisA=+Y  FollAlignAxisB=+Y  BaseAlignAxisB=+Z  RotationSequenceAxes=FollowerAxes  RotationSequence=XYX  RotationSequenceAngles=[0 0 0]  RotationSequenceAnglesUnits=deg  RotationMatrix=[1 0 0; 0 1 0; 0 0 1]
      settings: AttributesFormatString=|
      | %<RotationAngle> %<RotationAngleUnits>
      | about %<RotationStandardAxis>
  Rot2 : sm_lib/Frames and Transforms/Rigid Transform  TranslationMethod=None  TranslationStandardOffset=0  TranslationLengthUnit=m  TranslationStandardAxis=+Z  TranslationCartesianOffset=[0 0 0]  TranslationROffset=0  TranslationROffsetUnits=m  TranslationZOffset=0  TranslationZOffsetUnits=m  TranslationThetaOffset=0  TranslationThetaOffsetUnits=deg  RotationMethod=StandardAxis  RotationAngleUnits=deg  RotationStandardAxis=+Y  RotationAngle=90  RotationArbitraryAxis=[0 0 1]  FollAlignAxisA=+X  BaseAlignAxisA=+Y  FollAlignAxisB=+Y  BaseAlignAxisB=+Z  RotationSequenceAxes=FollowerAxes  RotationSequence=XYX  RotationSequenceAngles=[0 0 0]  RotationSequenceAnglesUnits=deg  RotationMatrix=[1 0 0; 0 1 0; 0 0 1]
      settings: AttributesFormatString=|
      | %<RotationAngle> %<RotationAngleUnits>
      | about %<RotationStandardAxis>
  Rot4 : sm_lib/Frames and Transforms/Rigid Transform  TranslationMethod=None  TranslationStandardOffset=0  TranslationLengthUnit=m  TranslationStandardAxis=+Z  TranslationCartesianOffset=[0 0 0]  TranslationROffset=0  TranslationROffsetUnits=m  TranslationZOffset=0  TranslationZOffsetUnits=m  TranslationThetaOffset=0  TranslationThetaOffsetUnits=deg  RotationMethod=StandardAxis  RotationAngleUnits=deg  RotationStandardAxis=+X  RotationAngle=90  RotationArbitraryAxis=[0 0 1]  FollAlignAxisA=+X  BaseAlignAxisA=+Y  FollAlignAxisB=+Y  BaseAlignAxisB=+Z  RotationSequenceAxes=FollowerAxes  RotationSequence=XYX  RotationSequenceAngles=[0 0 0]  RotationSequenceAnglesUnits=deg  RotationMatrix=[1 0 0; 0 1 0; 0 0 1]
      settings: AttributesFormatString=|
      | %<RotationAngle> %<RotationAngleUnits>
      | about %<RotationStandardAxis>
  Solid2 : sm_lib/Body Elements/Solid  InertiaType=CalculateFromGeometry  Mass=Robot1.Element1(1)  MassUnits=kg  CenterOfMass=[0 0 0]  CenterOfMassUnits=m  MomentsOfInertia=[1 1 1]  MomentsOfInertiaUnits=kg*m^2  ProductsOfInertia=[0 0 0]  ProductsOfInertiaUnits=kg*m^2  DensityBased=off  Density=1000  DensityUnits=kg/(m^3)  DoExposeReferenceFrame=on  SerializedFrames=<Frames/>  GraphicType=FromGeometry  MarkerShape=Sphere  MarkerSize=10  MarkerSizeUnits=m  GraphicVisPropType=SimpleVisualProperties  GraphicDiffuseColor=[0.6 0.0 0.0]  GraphicSpecularColor=[0.5 0.5 0.5 1.0]  GraphicAmbientColor=[0.15 0.15 0.15 1.0]  GraphicEmissiveColor=[0.0 0.0 0.0 1.0]  GraphicShininess=75  GraphicOpacity=1.0  GeometryShape=FromFile  RectangleSize=[1 1]  RectangleSizeUnits=m  BrickDimensions=[1 1 1]  BrickDimensionUnits=m  CylinderRadius=1  CylinderRadiusUnits=m  CylinderLength=1  CylinderLengthUnits=m  SphereRadius=1  SphereRadiusUnits=m  EllipsoidRadii=[1 1 1]  EllipsoidRadiiUnits=m  ExtrusionCrossSection=[1 1; -1 1; -1 -1; 1 -1]  ExtrusionCrossSectionUnits=m  ExtrusionLength=1  ExtrusionLengthUnits=m  PolygonNumSides=3  PolygonOuterRadius=1  PolygonOuterRadiusUnits=m  ExtGeomFileType=STEP  ExtGeomFileName=./StepData_DHPara/Element1.stp  ExtGeomFileUnits=m  RevolutionCrossSection=[1 1; 1 -1; 2 -1; 2 1]  RevolutionCrossSectionUnits=m  RevolutionExtent=Full  RevolutionAngle=180  RevolutionAngleUnits=deg
  Trans2 : sm_lib/Frames and Transforms/Rigid Transform  TranslationMethod=StandardAxis  TranslationStandardOffset=Robot1.Element1(2)  TranslationLengthUnit=m  TranslationStandardAxis=+Z  TranslationCartesianOffset=[0 0 0]  TranslationROffset=0  TranslationROffsetUnits=m  TranslationZOffset=0  TranslationZOffsetUnits=m  TranslationThetaOffset=0  TranslationThetaOffsetUnits=deg  RotationMethod=None  RotationAngleUnits=deg  RotationStandardAxis=+Z  RotationAngle=0.0  RotationArbitraryAxis=[0 0 1]  FollAlignAxisA=+X  BaseAlignAxisA=+Y  FollAlignAxisB=+Y  BaseAlignAxisB=+Z  RotationSequenceAxes=FollowerAxes  RotationSequence=XYX  RotationSequenceAngles=[0 0 0]  RotationSequenceAnglesUnits=deg  RotationMatrix=[1 0 0; 0 1 0; 0 0 1]
      settings: AttributesFormatString=|
      | %<TranslationStandardOffset> %<TranslationLengthUnit>
      | in %<TranslationStandardAxis>
  Trans3 : sm_lib/Frames and Transforms/Rigid Transform  TranslationMethod=StandardAxis  TranslationStandardOffset=Robot1.Element1(3)  TranslationLengthUnit=m  TranslationStandardAxis=+Z  TranslationCartesianOffset=[0 0 0]  TranslationROffset=0  TranslationROffsetUnits=m  TranslationZOffset=0  TranslationZOffsetUnits=m  TranslationThetaOffset=0  TranslationThetaOffsetUnits=deg  RotationMethod=None  RotationAngleUnits=deg  RotationStandardAxis=+Z  RotationAngle=0.0  RotationArbitraryAxis=[0 0 1]  FollAlignAxisA=+X  BaseAlignAxisA=+Y  FollAlignAxisB=+Y  BaseAlignAxisB=+Z  RotationSequenceAxes=FollowerAxes  RotationSequence=XYX  RotationSequenceAngles=[0 0 0]  RotationSequenceAnglesUnits=deg  RotationMatrix=[1 0 0; 0 1 0; 0 0 1]
      settings: AttributesFormatString=|
      | %<TranslationStandardOffset> %<TranslationLengthUnit>
      | in %<TranslationStandardAxis>
  B : PMIOPort  Port=1  Side=Left
  F : PMIOPort  Port=2  Side=Right
  connections:
  Rot4/RConn1 -- Solid2/RConn1
  Rot1/LConn1 -- Trans3/RConn1
  B/RConn1 -- Trans2/LConn1
  Rot2/LConn1 -- Trans2/RConn1
  Trans3/LConn1 -- Rot2/RConn1
  Rot1/RConn1 -- F/RConn1 -- Rot4/LConn1

== system Pong3D/Robot 1/Element2 ==
  Rot1 : sm_lib/Frames and Transforms/Rigid Transform  TranslationMethod=None  TranslationStandardOffset=0  TranslationLengthUnit=m  TranslationStandardAxis=+Z  TranslationCartesianOffset=[0 0 0]  TranslationROffset=0  TranslationROffsetUnits=m  TranslationZOffset=0  TranslationZOffsetUnits=m  TranslationThetaOffset=0  TranslationThetaOffsetUnits=deg  RotationMethod=StandardAxis  RotationAngleUnits=deg  RotationStandardAxis=+X  RotationAngle=90  RotationArbitraryAxis=[0 0 1]  FollAlignAxisA=+X  BaseAlignAxisA=+Y  FollAlignAxisB=+Y  BaseAlignAxisB=+Z  RotationSequenceAxes=FollowerAxes  RotationSequence=XYX  RotationSequenceAngles=[0 0 0]  RotationSequenceAnglesUnits=deg  RotationMatrix=[1 0 0; 0 1 0; 0 0 1]
      settings: AttributesFormatString=|
      | %<RotationAngle> %<RotationAngleUnits>
      | about %<RotationStandardAxis>
  Rot3 : sm_lib/Frames and Transforms/Rigid Transform  TranslationMethod=None  TranslationStandardOffset=0  TranslationLengthUnit=m  TranslationStandardAxis=+Z  TranslationCartesianOffset=[0 0 0]  TranslationROffset=0  TranslationROffsetUnits=m  TranslationZOffset=0  TranslationZOffsetUnits=m  TranslationThetaOffset=0  TranslationThetaOffsetUnits=deg  RotationMethod=StandardAxis  RotationAngleUnits=deg  RotationStandardAxis=-Y  RotationAngle=90  RotationArbitraryAxis=[0 0 1]  FollAlignAxisA=+X  BaseAlignAxisA=+Y  FollAlignAxisB=+Y  BaseAlignAxisB=+Z  RotationSequenceAxes=FollowerAxes  RotationSequence=XYX  RotationSequenceAngles=[0 0 0]  RotationSequenceAnglesUnits=deg  RotationMatrix=[1 0 0; 0 1 0; 0 0 1]
      settings: AttributesFormatString=|
      | %<RotationAngle> %<RotationAngleUnits>
      | about %<RotationStandardAxis>
  Rot4 : sm_lib/Frames and Transforms/Rigid Transform  TranslationMethod=None  TranslationStandardOffset=0  TranslationLengthUnit=m  TranslationStandardAxis=+Z  TranslationCartesianOffset=[0 0 0]  TranslationROffset=0  TranslationROffsetUnits=m  TranslationZOffset=0  TranslationZOffsetUnits=m  TranslationThetaOffset=0  TranslationThetaOffsetUnits=deg  RotationMethod=StandardAxis  RotationAngleUnits=deg  RotationStandardAxis=+Y  RotationAngle=90  RotationArbitraryAxis=[0 0 1]  FollAlignAxisA=+X  BaseAlignAxisA=+Y  FollAlignAxisB=+Y  BaseAlignAxisB=+Z  RotationSequenceAxes=FollowerAxes  RotationSequence=XYX  RotationSequenceAngles=[0 0 0]  RotationSequenceAnglesUnits=deg  RotationMatrix=[1 0 0; 0 1 0; 0 0 1]
      settings: AttributesFormatString=|
      | %<RotationAngle> %<RotationAngleUnits>
      | about %<RotationStandardAxis>
  Solid1 : sm_lib/Body Elements/Solid  InertiaType=PointMass  Mass=Robot1.Element2(1)  MassUnits=kg  CenterOfMass=[0 0 0]  CenterOfMassUnits=m  MomentsOfInertia=[1 1 1]  MomentsOfInertiaUnits=kg*m^2  ProductsOfInertia=[0 0 0]  ProductsOfInertiaUnits=kg*m^2  DensityBased=on  Density=1000  DensityUnits=kg/(m^3)  DoExposeReferenceFrame=on  SerializedFrames=<Frames/>  GraphicType=FromGeometry  MarkerShape=Sphere  MarkerSize=10  MarkerSizeUnits=m  GraphicVisPropType=SimpleVisualProperties  GraphicDiffuseColor=[1.0 0.0 0.0]  GraphicSpecularColor=[0.5 0.5 0.5 1.0]  GraphicAmbientColor=[0.15 0.15 0.15 1.0]  GraphicEmissiveColor=[0.0 0.0 0.0 1.0]  GraphicShininess=75  GraphicOpacity=1  GeometryShape=FromFile  RectangleSize=[1 1]  RectangleSizeUnits=m  BrickDimensions=[1 1 1]  BrickDimensionUnits=m  CylinderRadius=1  CylinderRadiusUnits=m  CylinderLength=1  CylinderLengthUnits=m  SphereRadius=1  SphereRadiusUnits=m  EllipsoidRadii=[1 1 1]  EllipsoidRadiiUnits=m  ExtrusionCrossSection=[1 1; -1 1; -1 -1; 1 -1]  ExtrusionCrossSectionUnits=m  ExtrusionLength=1  ExtrusionLengthUnits=m  PolygonNumSides=3  PolygonOuterRadius=1  PolygonOuterRadiusUnits=m  ExtGeomFileType=STEP  ExtGeomFileName=./StepData_DHPara/element2.stp  ExtGeomFileUnits=m  RevolutionCrossSection=[1 1; 1 -1; 2 -1; 2 1]  RevolutionCrossSectionUnits=m  RevolutionExtent=Full  RevolutionAngle=180  RevolutionAngleUnits=deg
  Trans3 : sm_lib/Frames and Transforms/Rigid Transform  TranslationMethod=StandardAxis  TranslationStandardOffset=Robot1.Element2(3)  TranslationLengthUnit=m  TranslationStandardAxis=+Z  TranslationCartesianOffset=[0 0 0]  TranslationROffset=0  TranslationROffsetUnits=m  TranslationZOffset=0  TranslationZOffsetUnits=m  TranslationThetaOffset=0  TranslationThetaOffsetUnits=deg  RotationMethod=None  RotationAngleUnits=deg  RotationStandardAxis=+Z  RotationAngle=0.0  RotationArbitraryAxis=[0 0 1]  FollAlignAxisA=+X  BaseAlignAxisA=+Y  FollAlignAxisB=+Y  BaseAlignAxisB=+Z  RotationSequenceAxes=FollowerAxes  RotationSequence=XYX  RotationSequenceAngles=[0 0 0]  RotationSequenceAnglesUnits=deg  RotationMatrix=[1 0 0; 0 1 0; 0 0 1]
      settings: AttributesFormatString=|
      | %<TranslationStandardOffset> %<TranslationLengthUnit>
      | in %<TranslationStandardAxis>
  B : PMIOPort  Port=1  Side=Left
  F : PMIOPort  Port=2  Side=Right
  connections:
  Rot3/RConn1 -- Rot1/LConn1 -- F/RConn1
  Trans3/LConn1 -- Rot4/RConn1
  Rot3/LConn1 -- Trans3/RConn1
  Rot4/LConn1 -- B/RConn1
  Rot1/RConn1 -- Solid1/RConn1
